simulink model "LUPA_MHKDR"  (R2023b)
settings: Solver=ode4  StartTime=0  StopTime=100  FixedStep=0.1  MaxStep=0.1  RelTol=1e-3
values from neighbouring files (symbols this model uses):
  ptoDampingLoss = -350    [wecSimInputFile.m]
undefined symbols (not defined in the file or in its folder): body, constraint, geometry, hydroData, mooring, pto
libraries: WECSim_Lib_Body_Elements x2, WECSim_Lib_Moorings x2, WECSim_Lib_Constraints x1, WECSim_Lib_Frames x1, dspindex x1, WECSim_Lib_PTOs x1
settings Model: Creator=Bosma  LastModifiedBy=mankleh
settings SolverCC: ZeroCrossControl=DisableAll  AlgebraicLoopSolver=TrustRegion  AutoInsertRateTranBlk=on
settings DataIOCC: ReturnWorkspaceOutputs=off
settings OptimizationCC: ReuseModelBlockBuffer=off  SimCompilerOptimization=on
settings DebuggingCC: UnconnectedInputMsg=warning  UnconnectedOutputMsg=warning  UnconnectedLineMsg=warning
settings ModelReferenceCC: EnableRefExpFcnMdlSchedulingChecks=on
settings RTWCC: DLArmComputeVersion=19.05

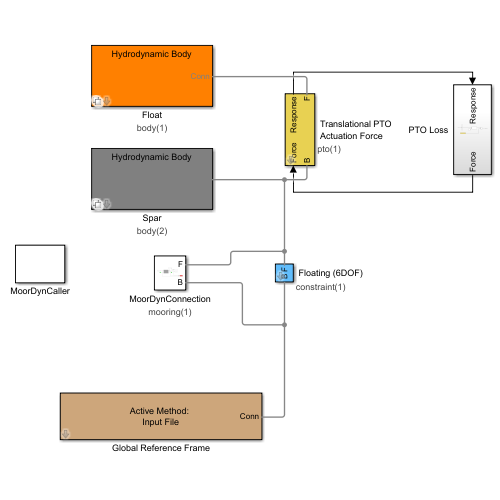
[thumbnail: Simulink's stored preview of the top-level diagram]
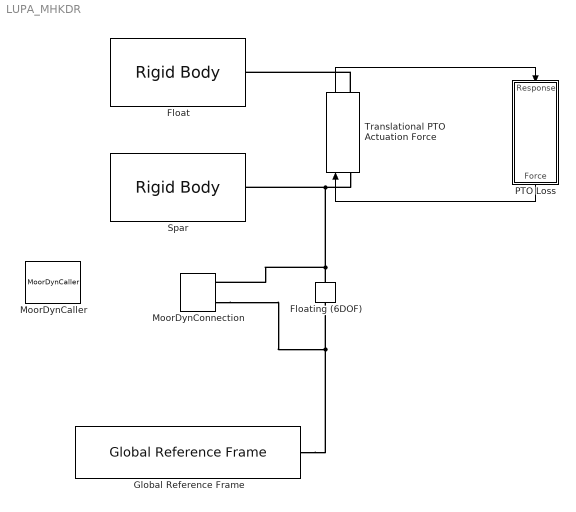
== system LUPA_MHKDR ==
  Float : WECSim_Lib_Body_Elements/Rigid Body  body=body(1)  h5File=hydroData/*.h5  geometryFile=geometry/*.stl  mass=0  inertia=0 0 0  inertiaProducts=0 0 0  nonHydro=0  nonlinearHydro=0  centerGravity=0 0 0  centerBuoyancy=0 0 0  dof=6  volume=0  QTFs=0  displacement=0 0 0  axis=0 1 0  angle=0  option=0  cd=0 0 0  ca=0 0 0  area=0 0 0  VME=0  rgME=0 0 0  z=0 0 1
  "Floating (6DOF) " : WECSim_Lib_Constraints/Floating (6DOF)  constraint=constraint(1)  loc="0  0  0"  displacement=0 0 0  y=0 1 0  z=0 0 1  upperLimitSpecify=off  upperLimitBound=0  upperLimitTransitionRegionWidth=0  upperLimitStiffness=0  upperLimitDamping=0  lowerLimitSpecify=off  lowerLimitBound=0  lowerLimitTransitionRegionWidth=0  lowerLimitStiffness=0  lowerLimitDamping=0
      settings: AttributesFormatString=%<constraint>
  Global Reference Frame : WECSim_Lib_Frames/Global Reference Frame  waves=waves  simu=simu  InputMethod=Input File  InputFile=wecSimInputFile.m  mode=normal  explorer=off  solver=ode4  startTime=0  rampTime=100  endTime=400  dt=0.1  cicEndTime=60  stateSpace=0  WaveClass=regular  height=2.5  period=8  elevationFile=NOT DEFINED  spectrumFile=NOT DEFINED  direction=0  spread=1  spectrumType=NOT DEFINED  phaseSeed=0  option=EqualEnergy
  MoorDynCaller : WECSim_Lib_Moorings/MoorDynCaller  simu=simu  mooring=mooring  numMoorDyn=0
  MoorDynConnection : WECSim_Lib_Moorings/MoorDynConnection  mooring=mooring(1)  MooringRef="0  0  0"  moorDynLines=0
      settings: AttributesFormatString=%<mooring>
  PTO Loss : Subsystem
  Spar : WECSim_Lib_Body_Elements/Rigid Body  body=body(2)  h5File=hydroData/*.h5  geometryFile=geometry/*.stl  mass=0  inertia=0 0 0  inertiaProducts=0 0 0  nonHydro=0  nonlinearHydro=0  centerGravity=0 0 0  centerBuoyancy=0 0 0  dof=6  volume=0  QTFs=0  displacement=0 0 0  axis=0 1 0  angle=0  option=0  cd=0 0 0  ca=0 0 0  area=0 0 0  VME=0  rgME=0 0 0  z=0 0 1
  "Translational PTO Actuation Force " : WECSim_Lib_PTOs/Translational PTO Actuation Force  pto=pto(1)  loc="0  0  0"  stiffness=0  damping=0  equilibriumPosition=0  pretension=0  displacement=0 0 0  y=0 1 0  z=0 0 1  upperLimitSpecify=off  upperLimitBound=0  upperLimitTransitionRegionWidth=0  upperLimitStiffness=0  upperLimitDamping=0  lowerLimitSpecify=off  lowerLimitBound=0  lowerLimitTransitionRegionWidth=0  lowerLimitStiffness=0  lowerLimitDamping=0
      settings: AttributesFormatString=%<pto>
  wires:
  "Translational PTO Actuation Force "/1 -> PTO Loss/1(Response)
  PTO Loss/1(Force) -> "Translational PTO Actuation Force "/1
  connections:
  "Translational PTO Actuation Force "/RConn1 -- Float/RConn1
  "Floating (6DOF) "/RConn1 -- "Translational PTO Actuation Force "/LConn1 -- Spar/RConn1 -- MoorDynConnection/LConn1
  Global Reference Frame/RConn1 -- MoorDynConnection/LConn2 -- "Floating (6DOF) "/LConn1

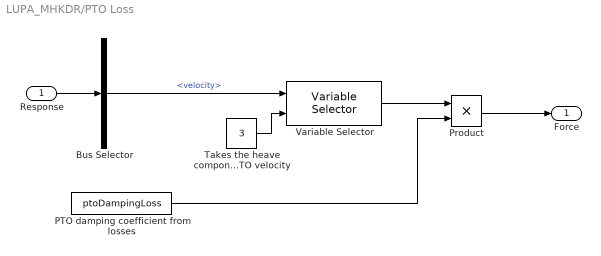
== system LUPA_MHKDR/PTO Loss ==
  Response : Inport
  Bus Selector : BusSelector  OutputSignals=velocity
  PTO damping coefficient from losses : Constant  Value=ptoDampingLoss
  Product : Product
  Takes the heave component of the PTO velocity : Constant  Value=3
  Variable Selector : dspindex/Variable Selector  NumInputs=1  rowsOrCols=Columns  IdxMode=Variable  Elements=[1 3]  ZerOneIdxMode=One-based  errmode=Clip Index  FillMode=on  FillValues=0
  Force : Outport
  wires:
  Response/1 -> Bus Selector/1
  Bus Selector/1 -> Variable Selector/1  "<velocity>"
  PTO damping coefficient from losses/1 -> Product/2
  Product/1 -> Force/1
  Variable Selector/1 -> Product/1
  Takes the heave component of the PTO velocity/1 -> Variable Selector/2
